simulink model "elastic_robot_arm_PID"  (R2018b)
settings: Solver=ode8  StartTime=0.0  StopTime=200  FixedStep=0.001  RelTol=1e-3
undefined symbols (not defined in the file or in its folder): sigbuilder_block
settings Model: Creator=TUAN HUA  LastModifiedBy=TUAN HUA

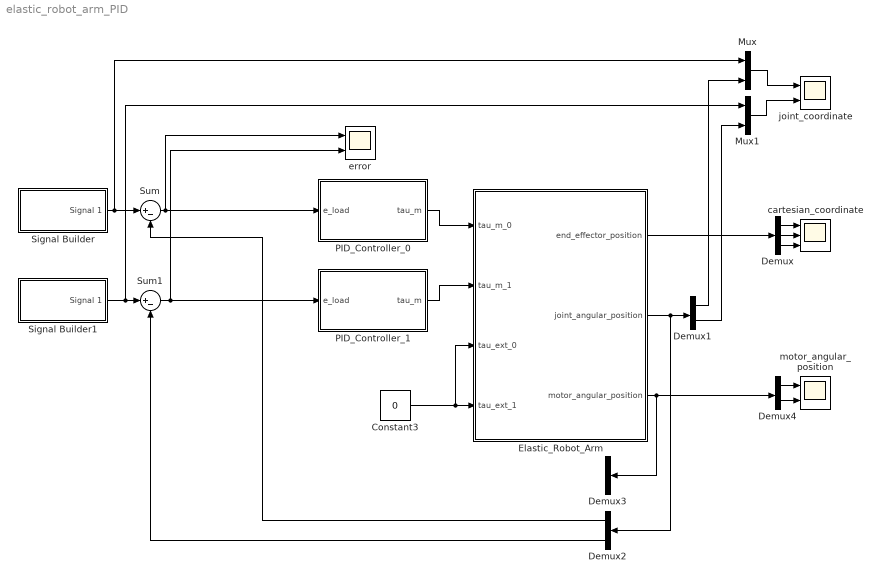
== system elastic_robot_arm_PID ==
  Constant3 : Constant  Value=0
  Demux : Demux  Outputs=3
  Demux{1..4} (4 alike) : Demux  Outputs=2
  Elastic_Robot_Arm : Subsystem
  Mux : Mux  Inputs=2
  Mux1 : Mux  Inputs=2
  PID_Controller_0 : Subsystem
  PID_Controller_1 : Subsystem
  Signal Builder : Subsystem  Tag=STV Subsys  LoadFcn=sigbuilder_block('load');  StartFcn=sigbuilder_block('start');  StopFcn=sigbuilder_block('stop');  ClipboardFcn=sigbuilder_block('clipboard');  mask(Sigbuilder block){tuvar=[0:10]}
      mask help: Simulink:masks:SigbuilderBlock_MD
      mask init:
      | if ~strcmp(get_param(bdroot(gcbh),'SimulationStatus'),'stopped') tuvar = sigbuilder_block('maskInit'); end
      settings: CopyFcn=sigbuilder_block('copy');  DeleteFcn=sigbuilder_block('delete');  ModelCloseFcn=sigbuilder_block('modelClose');  PreSaveFcn=sigbuilder_block('preSave');  PauseFcn=sigbuilder_block('pause');  ContinueFcn=sigbuilder_block('continue');  NameChangeFcn=sigbuilder_block('namechange');  OpenFcn=sigbuilder_block('open',[0 0 1024.5 518.25 ]);  CloseFcn=sigbuilder_block('close');
      mask Display: plot(0, 0, 100, 100,[2, 2, 32, 32, 2], [68, 8, 8, 68, 68],[32, 2], [38, 38], [32, 19, 2],[53, 60, 44], [32, 17, 17, 2],[16, 16, 31, 31]);txt = getActiveGroup(gcbh);text(2, 100, txt,'verticalAlignment', 'top');
  Signal Builder1 : Subsystem  Tag=STV Subsys  LoadFcn=sigbuilder_block('load');  StartFcn=sigbuilder_block('start');  StopFcn=sigbuilder_block('stop');  ClipboardFcn=sigbuilder_block('clipboard');  mask(Sigbuilder block){tuvar=[0:10]}
      mask help: Simulink:masks:SigbuilderBlock_MD
      mask init:
      | if ~strcmp(get_param(bdroot(gcbh),'SimulationStatus'),'stopped') tuvar = sigbuilder_block('maskInit'); end
      settings: CopyFcn=sigbuilder_block('copy');  DeleteFcn=sigbuilder_block('delete');  ModelCloseFcn=sigbuilder_block('modelClose');  PreSaveFcn=sigbuilder_block('preSave');  PauseFcn=sigbuilder_block('pause');  ContinueFcn=sigbuilder_block('continue');  NameChangeFcn=sigbuilder_block('namechange');  OpenFcn=sigbuilder_block('open',[6 0 1012.5 477.75 ]);  CloseFcn=sigbuilder_block('close');
      mask Display: plot(0, 0, 100, 100,[2, 2, 32, 32, 2], [68, 8, 8, 68, 68],[32, 2], [38, 38], [32, 19, 2],[53, 60, 44], [32, 17, 17, 2],[16, 16, 31, 31]);txt = getActiveGroup(gcbh);text(2, 100, txt,'verticalAlignment', 'top');
  Sum : Sum  Inputs=|+-
  Sum1 : Sum  Inputs=|+-
  cartesian_coordinate : Scope  NumInputPorts=3
  error : Scope  NumInputPorts=2
  joint_coordinate : Scope  NumInputPorts=2
  motor_angular_position : Scope  NumInputPorts=2
  wires:
  Constant3/1 -> Elastic_Robot_Arm/3(tau_ext_0), Elastic_Robot_Arm/4(tau_ext_1)
  Demux/3 -> cartesian_coordinate/3
  Demux/2 -> cartesian_coordinate/2
  Demux/1 -> cartesian_coordinate/1
  Elastic_Robot_Arm/1(end_effector_position) -> Demux/1
  Elastic_Robot_Arm/2(joint_angular_position) -> Demux1/1, Demux2/1
  Elastic_Robot_Arm/3(motor_angular_position) -> Demux3/1, Demux4/1
  Signal Builder/1(Signal 1) -> Mux/1, Sum/1
  Signal Builder1/1(Signal 1) -> Mux1/1, Sum1/1
  Demux4/1 -> motor_angular_position/1
  Demux4/2 -> motor_angular_position/2
  PID_Controller_0/1(tau_m) -> Elastic_Robot_Arm/1(tau_m_0)
  PID_Controller_1/1(tau_m) -> Elastic_Robot_Arm/2(tau_m_1)
  Sum1/1 -> PID_Controller_1/1(e_load), error/2
  Sum/1 -> PID_Controller_0/1(e_load), error/1
  Demux2/1 -> Sum/2
  Demux2/2 -> Sum1/2
  Demux1/1 -> Mux/2
  Demux1/2 -> Mux1/2
  Mux/1 -> joint_coordinate/1
  Mux1/1 -> joint_coordinate/2

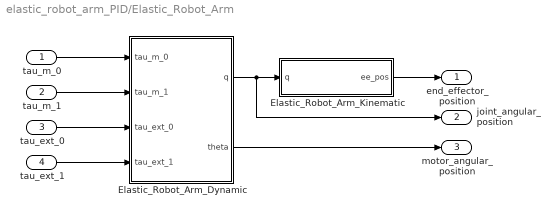
== system elastic_robot_arm_PID/Elastic_Robot_Arm ==
  tau_m_0 : Inport
  tau_m_1 : Inport  Port=2
  tau_ext_0 : Inport  Port=3
  tau_ext_1 : Inport  Port=4
  Elastic_Robot_Arm_Dynamic : Subsystem
  Elastic_Robot_Arm_Kinematic : Subsystem
  end_effector_position : Outport
  joint_angular_position : Outport  Port=2
  motor_angular_position : Outport  Port=3
  wires:
  Elastic_Robot_Arm_Dynamic/1(q) -> joint_angular_position/1, Elastic_Robot_Arm_Kinematic/1(q)
  tau_m_0/1 -> Elastic_Robot_Arm_Dynamic/1(tau_m_0)
  tau_m_1/1 -> Elastic_Robot_Arm_Dynamic/2(tau_m_1)
  tau_ext_0/1 -> Elastic_Robot_Arm_Dynamic/3(tau_ext_0)
  tau_ext_1/1 -> Elastic_Robot_Arm_Dynamic/4(tau_ext_1)
  Elastic_Robot_Arm_Kinematic/1(ee_pos) -> end_effector_position/1
  Elastic_Robot_Arm_Dynamic/2(theta) -> motor_angular_position/1

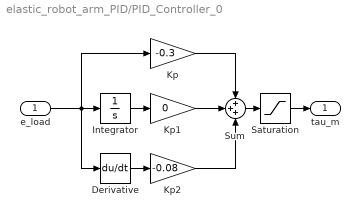
== system elastic_robot_arm_PID/PID_Controller_0 ==
  e_load : Inport
  Derivative : Derivative  CoefficientInTFapproximation=0
  Integrator : Integrator
  Kp : Gain  Gain=-0.3
  Kp1 : Gain  Gain=0
  Kp2 : Gain  Gain=-0.08
  Saturation : Saturate
  Sum : Sum  Inputs=+++
  tau_m : Outport
  wires:
  Saturation/1 -> tau_m/1
  Sum/1 -> Saturation/1
  Kp1/1 -> Sum/2
  Kp/1 -> Sum/1
  Kp2/1 -> Sum/3
  Integrator/1 -> Kp1/1
  Derivative/1 -> Kp2/1
  e_load/1 -> Derivative/1, Integrator/1, Kp/1

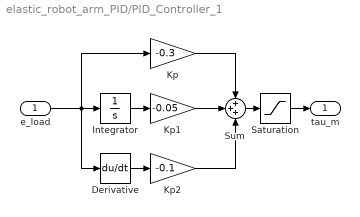
== system elastic_robot_arm_PID/PID_Controller_1 ==
  e_load : Inport
  Derivative : Derivative  CoefficientInTFapproximation=0
  Integrator : Integrator
  Kp : Gain  Gain=-0.3
  Kp1 : Gain  Gain=-0.05
  Kp2 : Gain  Gain=-0.1
  Saturation : Saturate
  Sum : Sum  Inputs=+++
  tau_m : Outport
  wires:
  e_load/1 -> Kp/1, Integrator/1, Derivative/1
  Derivative/1 -> Kp2/1
  Integrator/1 -> Kp1/1
  Kp2/1 -> Sum/3
  Kp/1 -> Sum/1
  Kp1/1 -> Sum/2
  Sum/1 -> Saturation/1
  Saturation/1 -> tau_m/1

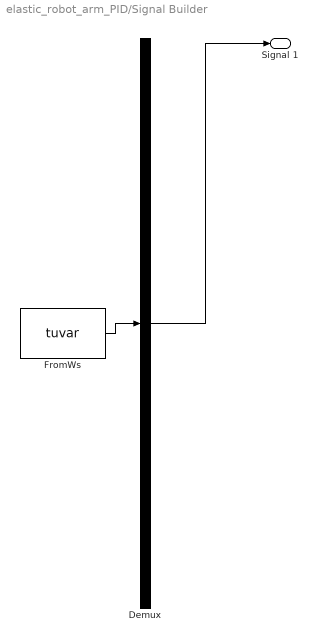
== system elastic_robot_arm_PID/Signal Builder ==
  Demux : Demux  Tag=STV Demux  Outputs=1
  FromWs : FromWorkspace  Tag=STV FromWs  VariableName=tuvar  SampleTime=0
      SigBuilderData=|
      | common.afterFinalStr = 'Extrapolate'
      | common.sampleTime = 0
      | dataSet.timeRange = [0 200]
      | dataSet.name = 'Group 1'
      | sbobj.Groups.Name = 'Group 1'
      | sbobj.Groups.Signals.Name = 'Signal 1'
      | sbobj.Groups.Signals.XData = [0 40 40 60 60 80.2 80.2 99.8 99.8 120 120 130 130 140 140 150 150 160.2 160.2 200]
      | sbobj.Groups.Signals.YData = [0.5 0.5 0 0 1 1 0 0 -0.5 -0.5 -1 -1 -0.5 -0.5 0 0 0.5 0.5 0 0]
      | sbobj.Groups.TimeRange = [0 200]
  Signal 1 : Outport  Tag=STV Outport
  wires:
  Demux/1 -> Signal 1/1
  FromWs/1 -> Demux/1

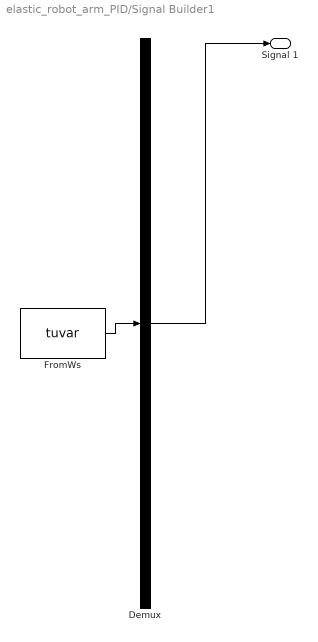
== system elastic_robot_arm_PID/Signal Builder1 ==
  Demux : Demux  Tag=STV Demux  Outputs=1
  FromWs : FromWorkspace  Tag=STV FromWs  VariableName=tuvar  SampleTime=0
      SigBuilderData=|
      | common.afterFinalStr = 'Extrapolate'
      | common.sampleTime = 0
      | dataSet.timeRange = [0 200]
      | dataSet.name = 'Group 1'
      | sbobj.Groups.Name = 'Group 1'
      | sbobj.Groups.Signals.Name = 'Signal 1'
      | sbobj.Groups.Signals.XData = [0 40 40 60 60 80 80 100 100 120 120 200]
      | sbobj.Groups.Signals.YData = [0.5 0.5 0 0 -0.5 -0.5 0 0 -0.5 -0.5 0 0]
      | sbobj.Groups.TimeRange = [0 200]
  Signal 1 : Outport  Tag=STV Outport
  wires:
  FromWs/1 -> Demux/1
  Demux/1 -> Signal 1/1

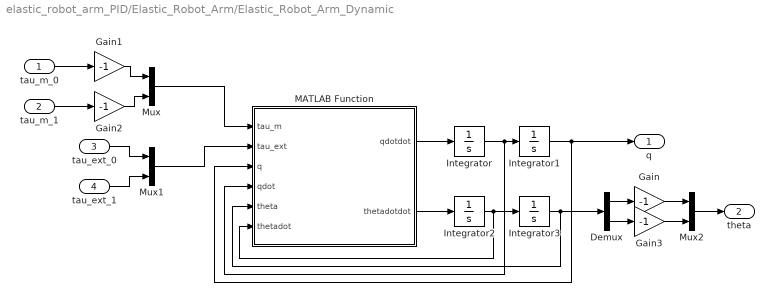
== system elastic_robot_arm_PID/Elastic_Robot_Arm/Elastic_Robot_Arm_Dynamic ==
  tau_m_0 : Inport
  tau_m_1 : Inport  Port=2
  tau_ext_0 : Inport  Port=3
  tau_ext_1 : Inport  Port=4
  Demux : Demux  Outputs=2
  Gain{,1..3} (4 alike) : Gain  Gain=-1
  Integrator{,1..3} (4 alike) : Integrator  InitialCondition=[0;0]
  MATLAB Function : MATLAB Function  TreatAsAtomicUnit=on
  Mux : Mux  Inputs=2
  Mux1 : Mux  Inputs=2
  Mux2 : Mux  Inputs=2
  q : Outport
  theta : Outport  Port=2
  wires:
  MATLAB Function/1(qdotdot) -> Integrator/1
  Integrator/1 -> MATLAB Function/4(qdot), Integrator1/1
  Integrator1/1 -> MATLAB Function/3(q), q/1
  MATLAB Function/2(thetadotdot) -> Integrator2/1
  Integrator2/1 -> Integrator3/1, MATLAB Function/6(thetadot)
  Integrator3/1 -> Demux/1, MATLAB Function/5(theta)
  tau_ext_0/1 -> Mux1/1
  tau_m_0/1 -> Gain1/1
  tau_ext_1/1 -> Mux1/2
  Mux1/1 -> MATLAB Function/2(tau_ext)
  Mux/1 -> MATLAB Function/1(tau_m)
  Gain1/1 -> Mux/1
  Mux2/1 -> theta/1
  Demux/1 -> Gain/1
  Gain/1 -> Mux2/1
  tau_m_1/1 -> Gain2/1
  Demux/2 -> Gain3/1
  Gain2/1 -> Mux/2
  Gain3/1 -> Mux2/2

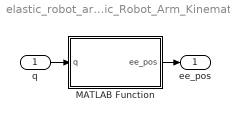
== system elastic_robot_arm_PID/Elastic_Robot_Arm/Elastic_Robot_Arm_Kinematic ==
  q : Inport
  MATLAB Function : MATLAB Function  TreatAsAtomicUnit=on
  ee_pos : Outport
  wires:
  q/1 -> MATLAB Function/1(q)
  MATLAB Function/1(ee_pos) -> ee_pos/1

== matlab function elastic_robot_arm_PID/Elastic_Robot_Arm/Elastic_Robot_Arm_Kinematic/MATLAB Function ==
  data: q input; ee_pos output
function ee_pos = kinematic(q)

    % Link length
    l0 = 0.1;
    l1 = 0.1;
    
    q_0 = q(1);
    q_1 = q(2);
    
    H2_0 = [[ cos(q_0)*cos(q_1), -sin(q_0), -cos(q_0)*sin(q_1), l1*cos(q_0)*cos(q_1)]
            [ cos(q_1)*sin(q_0),  cos(q_0), -sin(q_0)*sin(q_1), l1*cos(q_1)*sin(q_0)]
            [          sin(q_1),         0,           cos(q_1),     l0 + l1*sin(q_1)]
            [                 0,         0,                  0,                    1]];

    ee_pos = H2_0(1:3,4);

== matlab function elastic_robot_arm_PID/Elastic_Robot_Arm/Elastic_Robot_Arm_Dynamic/MATLAB Function ==
  data: tau_m input; tau_ext input; q input; qdot input; theta input; qdotdot output; thetadotdot output; thetadot input
function [qdotdot, thetadotdot] = dynamic(tau_m, tau_ext, q, qdot, theta, thetadot)
    % Link length
    l0 = 0.2;
    l1 = 0.2;
    % Link and motor mass
    ml0 = 0.5;
    ml1 = 0.5;
    mm0 = 0.3;
    mm1 = 0.3;
    % Link and motor inertia
    Ilxx0 = 0;
    Ilyy0 = 0;
    Ilzz0 = 0.065;
    Ilxx1 = 0;
    Ilyy1 = 0;
    Ilzz1 = 0.065;
    % Link and motor damping coefficient
    Dm0 = 0.06;
    Dm1 = 0.06;
    Dl0 = 0.006;
    Dl1 = 0.006;
    % Gravitational constant
    g = 9.81;
    % String stiffness
    K = 5;
    % Motor inertia matrix
    Im0 = 0.1;
    Im1 = 0.1;
    % Gear ratio
    N0 = 1;
    N1 = 1;
    
    q_0 = q(1);
    q_1 = q(2);
    qdot_0 = qdot(1);
    qdot_1 = qdot(2);
    
    % Mass matrix
    M = [[ Ilzz0 + Ilzz1 + (l1*l1*ml1)/4 - (l1*l1*ml1*sin(q_1)*sin(q_1))/4,                                                          0]
         [                                                             0, Ilyy1 + (l1*l1*ml1)/4 + Ilxx1*sin(q_0)*sin(q_0) - Ilyy1*sin(q_0)*sin(q_0)]];
    
    % Centrifugal and Coriolis forces
    C = zeros(2,1);
    
    C(1,1) = 0.5*(-(l1^2*ml1*sin(2*q_1))/2)*qdot_0*qdot_1 + 0.5*(-sin(2*q_0)*(Ilxx1 - Ilyy1))*qdot_1*qdot_1;
    C(2,1) = 0.5*((l1^2*ml1*sin(2*q_1))/4)*qdot_0*qdot_0 + 0.5*(2*sin(2*q_0)*(Ilxx1 - Ilyy1))*qdot_0*qdot_1;
    
    % Gravitational forces
    G = zeros(2,1);
    G(1,1) = 0;
    G(2,1) = ml1*g*(l1/2)*cos(q_1);

    % Dynamic equation in load side
    Dl = [Dl0,   0
            0, Dl1];
    tau_s = K*(theta - q);
    qdotdot = inv(M)*(tau_ext - C - G + tau_s - Dl*qdot);
    
    % Dynamic equation in motor side
    Dm = [Dm0,   0
            0, Dm1];
    B = [[Im0*(N0^2), 0]
         [         0, Im1*(N1^2)]];
    thetadotdot = inv(B)*(tau_m - tau_s - Dm*thetadot);
